simulink model "CSF_Model"  (R2022a)
settings: Solver=ode4  StartTime=0.0  StopTime=10000  FixedStep=0.01  MaxStep=0.1  MinStep=0.01  RelTol=1e-3  AbsTol=1e-6
undefined symbols (not defined in the file): b_EA, E_A0, E_C, E_IEG, E_SAS, E_V, E_VEN, f_ECS, f_SPI, k_m, P_ECS0, P_OLS, P_SLS, P_SPI0, P_SSS, pi_C0, pi_ECS0, Q_CSF, R_A0, R_AG, R_BBB, R_C0, R_CMC, R_CP, R_ECS, R_FM, R_IEGH, R_IEGL, R_PAS, R_PCS, R_PNS, R_SAS, R_SPI, R_V0, R_VEN, R_VEN0, sigbuilder_block, V_A0, V_Afree, V_BT_solid, V_C0, V_Cfree, V_ECS0, V_ICS0, V_PAS0, V_PNS0, V_SAS0, V_SPI0, V_T0, V_V0, V_VEN0, V_VEN_free, V_Vfree
libraries: cstblocks x8, dspstat3 x6, simulink x1
settings Model: SnapshotInterval=1  Creator=Administrator  LastModifiedBy=Administrator

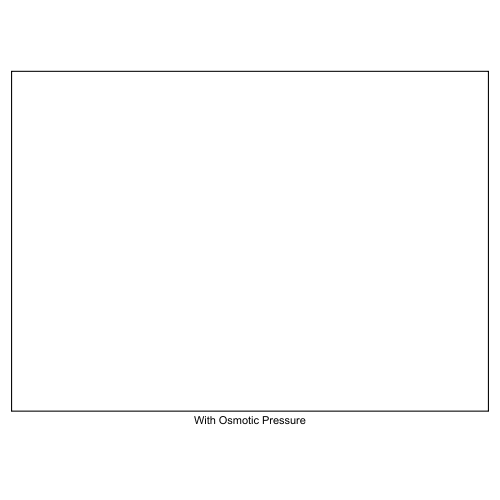
[thumbnail: Simulink's stored preview of the top-level diagram]
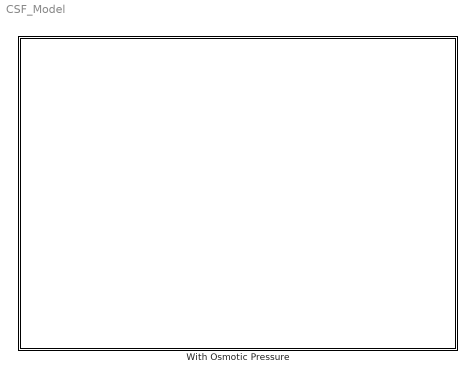
== system CSF_Model ==
  With Osmotic Pressure : Subsystem

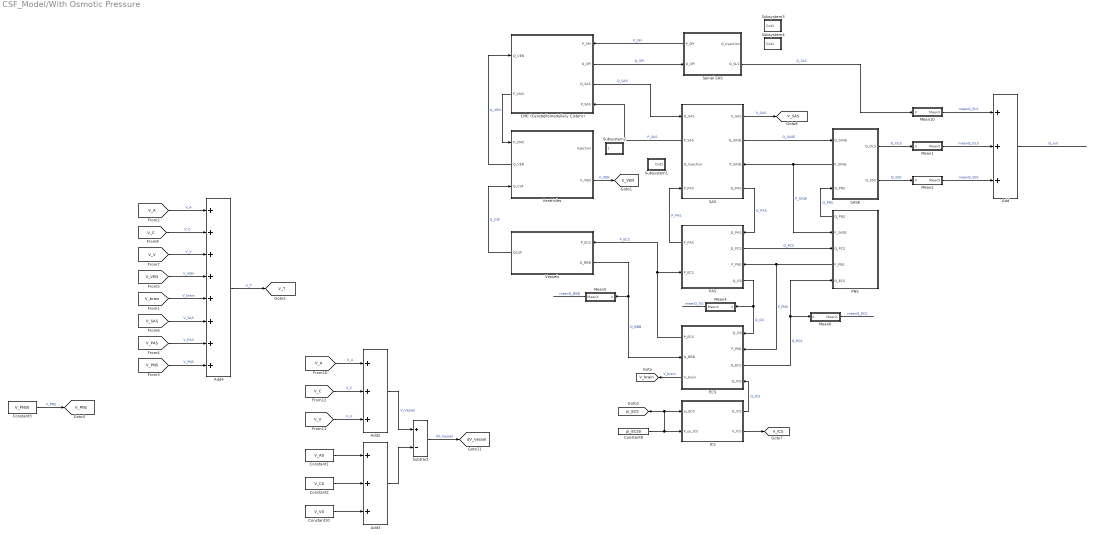
== system CSF_Model/With Osmotic Pressure ==
  Add : Sum  Inputs=+++
  Add2 : Sum  Inputs=+++
  Add3 : Sum  Inputs=+++
  Add4 : Sum  Inputs=++++++++
  CMC (Cerebellomedullary Cistern) : Subsystem
      settings: PortSchema="{\"entries\":[{\"content\":{\"sides\":[{\"content\":{\"connectorIds\":[\"In1\",\"Out3\"]},\"type\":\"ConnectorPlacement.EquallySpacedRectSide\",\"uuid\":\"013a87ed-5019-4cf7-bc7e-b763ecbf40be\"},{\"content\":{\"connectorIds\":[\"In2\",\"Out1\",\"Out2\",\"In3\"],\"side\":\"RIGHT\"},\"type\":\"ConnectorPlacement.EquallySpacedRectSide\",\"uuid\":\"57b2f7c1-58ac-4b82-ab5b-e050e476b33b\"},{\"content\":{\"connectorIds\":[],\"side\":\"TOP\"},\"type\":\"ConnectorPlacement.EquallySpacedRectSide\",\"uuid\":\"da2f9a82-30e0-49d1-9e6c-54ed808c9c6e\"}]},\"type\":\"ConnectorPlacement.EquallySpacedConnector\",\"uuid\":\"bd940c80-8986-43bc-ad7b-1b94db1ac316\"}],\"packageUris\":[\"http://schema.mathworks.com/mf0/Connector/R2020b\"],\"version\":\"1.0\"}"
  Constant1 : Constant  Value=V_A0
  Constant10 : Constant  Value=V_V0
  Constant2 : Constant  Value=V_C0
  Constant3 : Constant  Value=V_PNS0
  Constant8 : Constant  Value=pi_ECS0
  ECS : Subsystem
      settings: PortSchema="{\"entries\":[{\"content\":{\"sides\":[{\"content\":{\"connectorIds\":[\"Out2\",\"In1\",\"Out3\"]},\"type\":\"ConnectorPlacement.EquallySpacedRectSide\",\"uuid\":\"d1e0d4a5-d76a-43bf-98e1-ed8a33587d94\"},{\"content\":{\"connectorIds\":[\"In2\",\"Out1\",\"In3\",\"In4\"],\"side\":\"RIGHT\"},\"type\":\"ConnectorPlacement.EquallySpacedRectSide\",\"uuid\":\"a93046bb-1935-4fcc-a858-465d9e877f86\"},{\"content\":{\"connectorIds\":[],\"side\":\"TOP\"},\"type\":\"ConnectorPlacement.EquallySpacedRectSide\",\"uuid\":\"8ff1877f-8428-43f4-bdc2-a7f63dce98e3\"}]},\"type\":\"ConnectorPlacement.EquallySpacedConnector\",\"uuid\":\"3a5fbfdf-c4c7-43cd-80c3-39c50f2079ec\"}],\"packageUris\":[\"http://schema.mathworks.com/mf0/Connector/R2020b\"],\"version\":\"1.0\"}"
  ICS : Subsystem
  Mean1 : Subsystem
  Mean10 : Subsystem
  Mean2 : Subsystem
  Mean4 : Subsystem
  Mean5 : Subsystem
  Mean6 : Subsystem
  PAS : Subsystem
      settings: PortSchema="{\"entries\":[{\"content\":{\"sides\":[{\"content\":{\"connectorIds\":[\"Out3\",\"In1\"]},\"type\":\"ConnectorPlacement.EquallySpacedRectSide\",\"uuid\":\"c2f26e20-6fa7-4bf6-bac3-e1e4e9c4ec58\"},{\"content\":{\"connectorIds\":[\"In2\",\"Out1\",\"In3\",\"Out2\"],\"side\":\"RIGHT\"},\"type\":\"ConnectorPlacement.EquallySpacedRectSide\",\"uuid\":\"ae54b47a-8b10-42ee-b40e-b80c64c909c9\"},{\"content\":{\"connectorIds\":[],\"side\":\"TOP\"},\"type\":\"ConnectorPlacement.EquallySpacedRectSide\",\"uuid\":\"815b1455-9f59-434d-88b0-8812fa628978\"},{\"content\":{\"connectorIds\":[],\"side\":\"BOTTOM\"},\"type\":\"ConnectorPlacement.EquallySpacedRectSide\",\"uuid\":\"6b900877-34b4-4b91-99fd-dbb8757fe9e6\"}]},\"type\":\"ConnectorPlacement.EquallySpacedConnector\",\"uuid\":\"ecef9f3d-643d-4d92-8968-e42d0387bb2a\"}],\"packageUris\":[\"http://schema.mathworks.com/mf0/Connector/R2020b\"],\"version\":\"1.0\"}"
  PNS : Subsystem
      settings: PortSchema="{\"entries\":[{\"content\":{\"sides\":[{\"content\":{\"connectorIds\":[\"Out1\",\"In1\",\"In2\",\"Out2\",\"In3\"]},\"type\":\"ConnectorPlacement.EquallySpacedRectSide\",\"uuid\":\"5fbe6c9d-3498-4146-9f0b-b77779ec6dad\"},{\"content\":{\"connectorIds\":[],\"side\":\"RIGHT\"},\"type\":\"ConnectorPlacement.EquallySpacedRectSide\",\"uuid\":\"fbf01b15-7a9f-409e-af5d-c73289629c2f\"},{\"content\":{\"connectorIds\":[],\"side\":\"TOP\"},\"type\":\"ConnectorPlacement.EquallySpacedRectSide\",\"uuid\":\"84a27698-b118-4183-ac33-cd71cc4704df\"}]},\"type\":\"ConnectorPlacement.EquallySpacedConnector\",\"uuid\":\"3a25198c-4299-4e36-a61d-eed86b0dea68\"}],\"packageUris\":[\"http://schema.mathworks.com/mf0/Connector/R2020b\"],\"version\":\"1.0\"}"
  SAS : Subsystem
      settings: PortSchema="{\"entries\":[{\"content\":{\"sides\":[{\"content\":{\"connectorIds\":[\"In1\",\"Out4\",\"In2\",\"In3\"]},\"type\":\"ConnectorPlacement.EquallySpacedRectSide\",\"uuid\":\"ca5be0dd-e4d9-4d74-8ff5-165f520bee20\"},{\"content\":{\"connectorIds\":[\"Out1\",\"Out2\",\"In4\",\"Out3\"],\"side\":\"RIGHT\"},\"type\":\"ConnectorPlacement.EquallySpacedRectSide\",\"uuid\":\"d1bc81c7-8cba-48bb-8bc1-5472ec1443ad\"},{\"content\":{\"connectorIds\":[],\"side\":\"TOP\"},\"type\":\"ConnectorPlacement.EquallySpacedRectSide\",\"uuid\":\"685eba57-22e9-4397-b0db-5008f2d3101d\"}]},\"type\":\"ConnectorPlacement.EquallySpacedConnector\",\"uuid\":\"2486ab90-8cac-42ad-9c36-b2644eb474f8\"}],\"packageUris\":[\"http://schema.mathworks.com/mf0/Connector/R2020b\"],\"version\":\"1.0\"}"
  SASE : Subsystem
      settings: PortSchema="{\"entries\":[{\"content\":{\"sides\":[{\"content\":{\"connectorIds\":[\"In1\",\"Out3\",\"In2\"]},\"type\":\"ConnectorPlacement.EquallySpacedRectSide\",\"uuid\":\"73239018-6b84-4d1b-a39c-7360c9503bc6\"},{\"content\":{\"connectorIds\":[\"Out1\",\"Out2\"],\"side\":\"RIGHT\"},\"type\":\"ConnectorPlacement.EquallySpacedRectSide\",\"uuid\":\"b723cfc7-fedc-421a-9fba-aa0734355de6\"},{\"content\":{\"connectorIds\":[],\"side\":\"TOP\"},\"type\":\"ConnectorPlacement.EquallySpacedRectSide\",\"uuid\":\"de4b320f-3afa-4cf6-aa90-abae206980c0\"}]},\"type\":\"ConnectorPlacement.EquallySpacedConnector\",\"uuid\":\"1ba6b848-2c16-4613-b6b1-fdcb918bcf69\"}],\"packageUris\":[\"http://schema.mathworks.com/mf0/Connector/R2020b\"],\"version\":\"1.0\"}"
  Spinal SAS : Subsystem
      settings: PortSchema="{\"entries\":[{\"content\":{\"sides\":[{\"content\":{\"connectorIds\":[\"Out2\",\"In1\"]},\"type\":\"ConnectorPlacement.EquallySpacedRectSide\",\"uuid\":\"013a87ed-5019-4cf7-bc7e-b763ecbf40be\"},{\"content\":{\"connectorIds\":[\"In2\",\"Out1\"],\"side\":\"RIGHT\"},\"type\":\"ConnectorPlacement.EquallySpacedRectSide\",\"uuid\":\"57b2f7c1-58ac-4b82-ab5b-e050e476b33b\"},{\"content\":{\"connectorIds\":[],\"side\":\"TOP\"},\"type\":\"ConnectorPlacement.EquallySpacedRectSide\",\"uuid\":\"da2f9a82-30e0-49d1-9e6c-54ed808c9c6e\"}]},\"type\":\"ConnectorPlacement.EquallySpacedConnector\",\"uuid\":\"bd940c80-8986-43bc-ad7b-1b94db1ac316\"}],\"packageUris\":[\"http://schema.mathworks.com/mf0/Connector/R2020b\"],\"version\":\"1.0\"}"
  Subsystem1 : Subsystem
  Subsystem2 : Subsystem
  Subsystem3 : Subsystem
  Subsystem4 : Subsystem
  Subtract : Sum  Inputs=+-
  Ventricles : Subsystem
      settings: PortSchema="{\"entries\":[{\"content\":{\"sides\":[{\"content\":{\"connectorIds\":[\"In1\",\"Out2\",\"In2\"]},\"type\":\"ConnectorPlacement.EquallySpacedRectSide\",\"uuid\":\"013a87ed-5019-4cf7-bc7e-b763ecbf40be\"},{\"content\":{\"connectorIds\":[\"In3\",\"Out1\"],\"side\":\"RIGHT\"},\"type\":\"ConnectorPlacement.EquallySpacedRectSide\",\"uuid\":\"57b2f7c1-58ac-4b82-ab5b-e050e476b33b\"},{\"content\":{\"connectorIds\":[],\"side\":\"TOP\"},\"type\":\"ConnectorPlacement.EquallySpacedRectSide\",\"uuid\":\"da2f9a82-30e0-49d1-9e6c-54ed808c9c6e\"}]},\"type\":\"ConnectorPlacement.EquallySpacedConnector\",\"uuid\":\"bd940c80-8986-43bc-ad7b-1b94db1ac316\"}],\"packageUris\":[\"http://schema.mathworks.com/mf0/Connector/R2020b\"],\"version\":\"1.0\"}"
  Vessels : Subsystem
      settings: PortSchema="{\"entries\":[{\"content\":{\"sides\":[{\"content\":{\"connectorIds\":[\"Out2\"]},\"type\":\"ConnectorPlacement.EquallySpacedRectSide\",\"uuid\":\"02216f8d-b656-405c-ace7-fa57996d1b51\"},{\"content\":{\"connectorIds\":[\"In1\",\"Out1\"],\"side\":\"RIGHT\"},\"type\":\"ConnectorPlacement.EquallySpacedRectSide\",\"uuid\":\"1efca463-a03b-437d-a556-a9f9cadbd1b9\"},{\"content\":{\"connectorIds\":[],\"side\":\"TOP\"},\"type\":\"ConnectorPlacement.EquallySpacedRectSide\",\"uuid\":\"405cde4e-e8e7-4444-912c-c8c68c2302e6\"}]},\"type\":\"ConnectorPlacement.EquallySpacedConnector\",\"uuid\":\"ec00ee8b-baba-493b-8b97-ad2027431ac2\"}],\"packageUris\":[\"http://schema.mathworks.com/mf0/Connector/R2020b\"],\"version\":\"1.0\"}"
  tag scope: V_ICS=global, V_PNS=global, V_SAS=global, V_T=global, V_VEN=global, V_brain=global, dV_Vessel=global, pi_ECS=global
  wires:
  SAS/1(V_SAS) -> [V_SAS]  "V_SAS"
  Mean1/1(MeanX) -> Add/2  "meanQ_OLS"
  ECS/2(V_brain) -> [V_brain]  "V_brain"
  ICS/1(Q_ICS) -> ECS/2(Q_ICS)  "Q_ICS"
  ICS/2(V_ICS) -> [V_ICS]
  SASE/2(Q_SSS) -> Mean2/1(X)  "Q_SSS"
  Mean2/1(MeanX) -> Add/3  "meanQ_SSS"
  ECS/3(P_ECS) -> PAS/1(P_ECS), Vessels/1(P_ECS)  "P_ECS"
  ECS/1(Q_ECS) -> Mean6/1(X), PNS/3(Q_ECS)  "Q_ECS"
  SASE/1(Q_OLS) -> Mean1/1(X)  "Q_OLS"
  PAS/3(P_PAS) -> SAS/3(P_PAS)  "P_PAS"
  PNS/1(Q_PNS) -> SASE/2(Q_PNS)  "Q_PNS"
  PAS/2(Q_GS) -> Mean4/1(X), ECS/4(Q_GS)  "Q_GS"
  PNS/2(P_PNS) -> ECS/3(P_PNS), PAS/3(P_PNS)  "P_PNS"
  PAS/1(Q_PCS) -> PNS/2(Q_PCS)  "Q_PCS"
  Ventricles/1(V_VEN) -> [V_VEN]  "V_VEN"
  SASE/3(P_SASE) -> PNS/1(P_SASE), SAS/4(P_SASE)  "P_SASE"
  Add/1 -> ?  "Q_out"
  Mean6/1(MeanX) -> ?  "meanQ_ECS"
  Constant8/1 -> [pi_ECS], ICS/1(pi_ECS), ICS/2(P_os_ICS)
  Vessels/1(Q_BBB) -> ECS/1(Q_BBB), Mean5/1(X)  "Q_BBB"
  Vessels/2(QCSF) -> Ventricles/2(Q_CSF)  "Q_CSF"
  Spinal SAS/1(Q_SLS) -> Mean10/1(X)  "Q_SLS"
  Mean10/1(MeanX) -> Add/1  "meanQ_SLS"
  SAS/4(P_SAS) -> CMC (Cerebellomedullary Cistern)/3(P_SAS)  "P_SAS"
  CMC (Cerebellomedullary Cistern)/2(Q_SAS) -> SAS/1(Q_SAS)  "Q_SAS"
  Add4/1 -> [V_T]  "V_T"
  [V_C] -> Add4/2  "V_C"
  [V_SAS] -> Add4/6  "V_SAS"
  [V_VEN] -> Add4/4  "V_VEN"
  [V_V] -> Add4/3  "V_V"
  [V_PNS] -> Add4/8  "V_PNS"
  [V_A] -> Add4/1  "V_A"
  [V_brain] -> Add4/5  "V_brain"
  [V_PAS] -> Add4/7  "V_PAS"
  Mean4/1(MeanX) -> ?  "meanQ_GS"
  SAS/3(Q_PAS) -> PAS/2(Q_PAS)  "Q_PAS"
  SAS/2(Q_SASE) -> SASE/1(Q_SASE)  "Q_SASE"
  Mean5/1(MeanX) -> ?  "meanQ_BBB"
  Constant3/1 -> [V_PNS]  "V_PNS"
  Spinal SAS/2(P_SPI) -> CMC (Cerebellomedullary Cistern)/2(P_SPI)  "P_SPI"
  CMC (Cerebellomedullary Cistern)/1(Q_SPI) -> Spinal SAS/1(Q_SPI)  "Q_SPI"
  [V_C] -> Add2/2  "V_C"
  [V_V] -> Add2/3  "V_V"
  [V_A] -> Add2/1  "V_A"
  Constant1/1 -> Add3/1
  Constant2/1 -> Add3/2
  Constant10/1 -> Add3/3
  Subtract/1 -> [dV_Vessel]  "dV_Vessel"
  Add2/1 -> Subtract/1  "V_Vessel"
  Add3/1 -> Subtract/2
  Ventricles/2(Q_VEN) -> CMC (Cerebellomedullary Cistern)/1(Q_VEN)  "Q_VEN"
  CMC (Cerebellomedullary Cistern)/3(P_CMC) -> Ventricles/1(P_CMC)

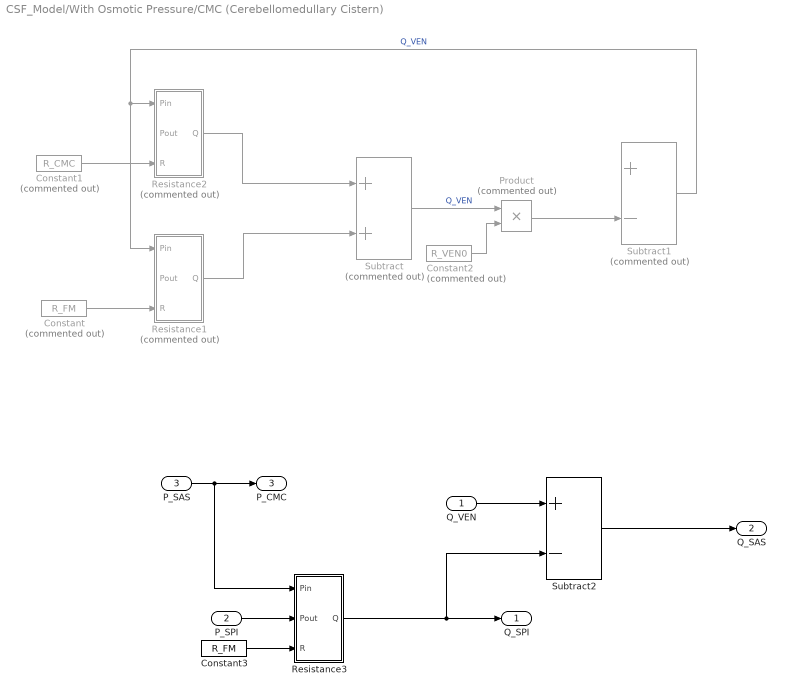
== system CSF_Model/With Osmotic Pressure/CMC (Cerebellomedullary Cistern) ==
  Q_VEN : Inport
  P_SPI : Inport  Port=2
  P_SAS : Inport  Port=3
  Constant : Constant  Commented=on  Value=R_FM
  Constant1 : Constant  Commented=on  Value=R_CMC
  Constant2 : Constant  Commented=on  Value=R_VEN0
  Constant3 : Constant  Value=R_FM
  Product : Product  Commented=on
  Resistance1 : Subsystem  Commented=on
  Resistance2 : Subsystem  Commented=on
  Resistance3 : Subsystem
  Subtract : Sum  Commented=on
  Subtract1 : Sum  Commented=on  Inputs=+-
  Subtract2 : Sum  Inputs=+-
  Q_SPI : Outport
  Q_SAS : Outport  Port=2
  P_CMC : Outport  Port=3
  wires:
  Constant/1 -> Resistance1/3(R)
  Resistance1/1(Q) -> Subtract/2
  Constant1/1 -> Resistance2/3(R)
  Resistance2/1(Q) -> Subtract/1
  Subtract/1 -> Product/1  "Q_VEN"
  Constant2/1 -> Product/2
  Product/1 -> Subtract1/2
  Subtract1/1 -> Resistance1/1(Pin), Resistance2/1(Pin)  "Q_VEN"
  P_SAS/1 -> Resistance3/1(Pin), P_CMC/1
  P_SPI/1 -> Resistance3/2(Pout)
  Constant3/1 -> Resistance3/3(R)
  Resistance3/1(Q) -> Subtract2/2, Q_SPI/1
  Q_VEN/1 -> Subtract2/1
  Subtract2/1 -> Q_SAS/1

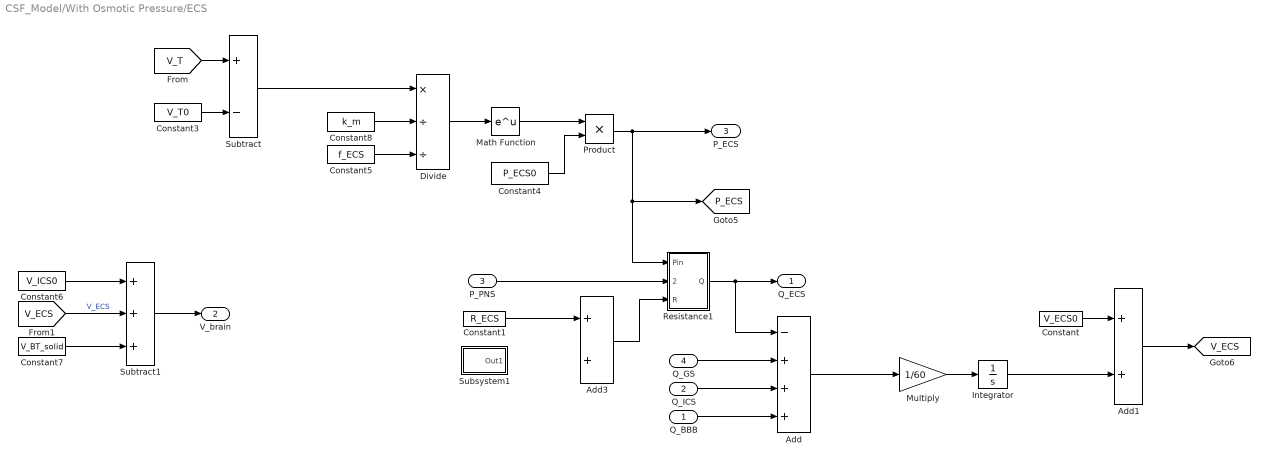
== system CSF_Model/With Osmotic Pressure/ECS ==
  Q_BBB : Inport
  Q_ICS : Inport  Port=2
  P_PNS : Inport  Port=3
  Q_GS : Inport  Port=4
  Add : Sum  Inputs=-+++
  Add1 : Sum
  Add3 : Sum
  Constant : Constant  Value=V_ECS0
  Constant1 : Constant  Value=R_ECS
  Constant3 : Constant  Value=V_T0
  Constant4 : Constant  Value=P_ECS0
  Constant5 : Constant  Value=f_ECS
  Constant6 : Constant  Value=V_ICS0
  Constant7 : Constant  Value=V_BT_solid
  Constant8 : Constant  Value=k_m
  Divide : Product  Inputs=*//
  Integrator : Integrator
  Math Function : Math
  Multiply : Gain  Gain=1/60
  Product : Product
  Resistance1 : Subsystem
  Subsystem1 : Subsystem
  Subtract : Sum  Inputs=+-
  Subtract1 : Sum  Inputs=+++
  Q_ECS : Outport
  V_brain : Outport  Port=2
  P_ECS : Outport  Port=3
  tag scope: P_ECS=global, V_ECS=global
  wires:
  Add3/1 -> Resistance1/3(R)
  Resistance1/1(Q) -> Add/1, Q_ECS/1
  Constant1/1 -> Add3/1
  P_PNS/1 -> Resistance1/2(Pout)
  Add1/1 -> [V_ECS]
  Add/1 -> Multiply/1
  Q_ICS/1 -> Add/3
  Q_GS/1 -> Add/2
  Product/1 -> Resistance1/1(Pin), [P_ECS], P_ECS/1
  Q_BBB/1 -> Add/4
  Multiply/1 -> Integrator/1
  Constant5/1 -> Divide/3
  Constant8/1 -> Divide/2
  Math Function/1 -> Product/1
  Divide/1 -> Math Function/1
  Constant4/1 -> Product/2
  Integrator/1 -> Add1/2
  Constant/1 -> Add1/1
  [V_T] -> Subtract/1
  Constant3/1 -> Subtract/2
  Constant6/1 -> Subtract1/1
  [V_ECS] -> Subtract1/2  "V_ECS"
  Subtract1/1 -> V_brain/1
  Constant7/1 -> Subtract1/3
  Subtract/1 -> Divide/1

== system CSF_Model/With Osmotic Pressure/ICS ==
  pi_ECS : Inport
  P_os_ICS : Inport  Port=2
  Add : Sum
  Constant2 : Constant  Value=V_ICS0
  Constant3 : Constant
  Integrator : Integrator
  Multiply : Gain  Gain=-1
  Multiply1 : Gain  Gain=-1
  Multiply2 : Gain  Gain=-1
  Resistance1 : Subsystem
  Q_ICS : Outport
  V_ICS : Outport  Port=2
  wires:
  Add/1 -> V_ICS/1
  Constant2/1 -> Add/2
  Integrator/1 -> Add/1
  Multiply/1 -> Integrator/1
  Resistance1/1(Q) -> Q_ICS/1, Multiply/1
  pi_ECS/1 -> Multiply1/1
  P_os_ICS/1 -> Multiply2/1
  Multiply1/1 -> Resistance1/1(Pin)
  Multiply2/1 -> Resistance1/2(Pout)
  Constant3/1 -> Resistance1/3(R)

== system CSF_Model/With Osmotic Pressure/Mean1 ==
  X : Inport
  Constant : Constant  Value=0.1
  Moving Average : dspstat3/Moving Average  Method=Sliding window  ForgettingFactorPort=off  SpecifyWindowLength=on  WindowLength=1  ForgettingFactor=0.9  SimulateUsing=Code generation
  Product : Product
  Step : Step  Time=10  SampleTime=0
  Varying Lowpass Filter : cstblocks/Linear Parameter Varying/Varying Lowpass Filter  N=1
  MeanX : Outport
  wires:
  Constant/1 -> Varying Lowpass Filter/2
  X/1 -> Product/2
  Moving Average/1 -> Varying Lowpass Filter/1
  Product/1 -> Moving Average/1
  Step/1 -> Product/1
  Varying Lowpass Filter/1 -> MeanX/1

== system CSF_Model/With Osmotic Pressure/Mean10 ==
  X : Inport
  Constant : Constant  Value=0.1
  Moving Average : dspstat3/Moving Average  Method=Sliding window  ForgettingFactorPort=off  SpecifyWindowLength=on  WindowLength=1  ForgettingFactor=0.9  SimulateUsing=Code generation
  Product : Product
  Step : Step  Time=10  SampleTime=0
  Varying Lowpass Filter : cstblocks/Linear Parameter Varying/Varying Lowpass Filter  N=1
  MeanX : Outport
  wires:
  Constant/1 -> Varying Lowpass Filter/2
  X/1 -> Product/2
  Moving Average/1 -> Varying Lowpass Filter/1
  Product/1 -> Moving Average/1
  Step/1 -> Product/1
  Varying Lowpass Filter/1 -> MeanX/1

== system CSF_Model/With Osmotic Pressure/Mean2 ==
  X : Inport
  Constant : Constant  Value=0.1
  Moving Average : dspstat3/Moving Average  Method=Sliding window  ForgettingFactorPort=off  SpecifyWindowLength=on  WindowLength=1  ForgettingFactor=0.9  SimulateUsing=Code generation
  Product : Product
  Step : Step  Time=10  SampleTime=0
  Varying Lowpass Filter : cstblocks/Linear Parameter Varying/Varying Lowpass Filter  N=1
  MeanX : Outport
  wires:
  Constant/1 -> Varying Lowpass Filter/2
  X/1 -> Product/2
  Moving Average/1 -> Varying Lowpass Filter/1
  Product/1 -> Moving Average/1
  Step/1 -> Product/1
  Varying Lowpass Filter/1 -> MeanX/1

== system CSF_Model/With Osmotic Pressure/Mean4 ==
  X : Inport
  Constant : Constant  Value=0.1
  Constant1 : Constant  Value=0.1
  Moving Average1 : dspstat3/Moving Average  Method=Sliding window  ForgettingFactorPort=off  SpecifyWindowLength=on  WindowLength=1  ForgettingFactor=0.9  SimulateUsing=Code generation
  Product : Product
  Step : Step  Time=10  SampleTime=0
  Varying Lowpass Filter : cstblocks/Linear Parameter Varying/Varying Lowpass Filter  N=1
  Varying Lowpass Filter1 : cstblocks/Linear Parameter Varying/Varying Lowpass Filter  N=1
  MeanX : Outport
  wires:
  Constant/1 -> Varying Lowpass Filter/2
  X/1 -> Product/2
  Product/1 -> Moving Average1/1
  Step/1 -> Product/1
  Varying Lowpass Filter/1 -> Varying Lowpass Filter1/1
  Moving Average1/1 -> Varying Lowpass Filter/1
  Constant1/1 -> Varying Lowpass Filter1/2
  Varying Lowpass Filter1/1 -> MeanX/1

== system CSF_Model/With Osmotic Pressure/Mean5 ==
  X : Inport
  Constant : Constant  Value=0.1
  Moving Average : dspstat3/Moving Average  Method=Sliding window  ForgettingFactorPort=off  SpecifyWindowLength=on  WindowLength=1  ForgettingFactor=0.9  SimulateUsing=Code generation
  Product : Product
  Step : Step  Time=10  SampleTime=0
  Varying Lowpass Filter : cstblocks/Linear Parameter Varying/Varying Lowpass Filter  N=1
  MeanX : Outport
  wires:
  Constant/1 -> Varying Lowpass Filter/2
  X/1 -> Product/2
  Moving Average/1 -> Varying Lowpass Filter/1
  Product/1 -> Moving Average/1
  Step/1 -> Product/1
  Varying Lowpass Filter/1 -> MeanX/1

== system CSF_Model/With Osmotic Pressure/Mean6 ==
  X : Inport
  Constant : Constant  Value=0.1
  Moving Average : dspstat3/Moving Average  Method=Sliding window  ForgettingFactorPort=off  SpecifyWindowLength=on  WindowLength=1  ForgettingFactor=0.9  SimulateUsing=Code generation
  Product : Product
  Step : Step  Time=10  SampleTime=0
  Varying Lowpass Filter : cstblocks/Linear Parameter Varying/Varying Lowpass Filter  N=1
  MeanX : Outport
  wires:
  Constant/1 -> Varying Lowpass Filter/2
  X/1 -> Product/2
  Moving Average/1 -> Varying Lowpass Filter/1
  Product/1 -> Moving Average/1
  Step/1 -> Product/1
  Varying Lowpass Filter/1 -> MeanX/1

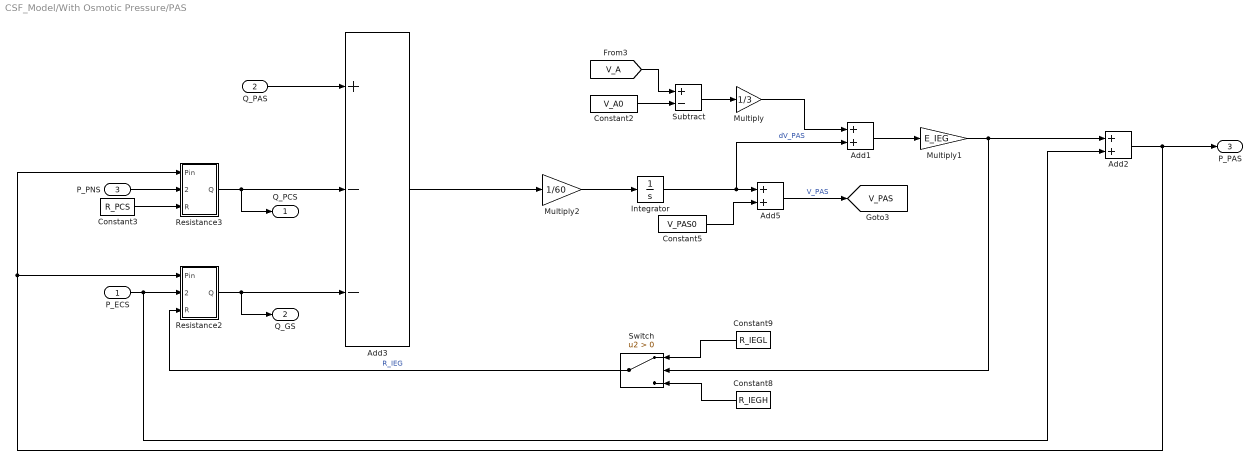
== system CSF_Model/With Osmotic Pressure/PAS ==
  P_ECS : Inport
  Q_PAS : Inport  Port=2
  P_PNS : Inport  Port=3
  Add1 : Sum
  Add2 : Sum
  Add3 : Sum  Inputs=+--
  Add5 : Sum
  Constant2 : Constant  Value=V_A0
  Constant3 : Constant  Value=R_PCS
  Constant5 : Constant  Value=V_PAS0
  Constant8 : Constant  Value=R_IEGH
  Constant9 : Constant  Value=R_IEGL
  Integrator : Integrator
  Multiply : Gain  Gain=1/3
  Multiply1 : Gain  Gain=E_IEG
  Multiply2 : Gain  Gain=1/60
  Resistance2 : Subsystem
  Resistance3 : Subsystem
  Subtract : Sum  Inputs=+-
  Switch : Switch  Criteria=u2 > Threshold  SaturateOnIntegerOverflow=off  InputSameDT=off
  Q_PCS : Outport
  Q_GS : Outport  Port=2
  P_PAS : Outport  Port=3
  tag scope: V_PAS=global
  wires:
  Multiply1/1 -> Switch/2, Add2/1
  Constant9/1 -> Switch/1
  Resistance2/1(Q) -> Add3/3, Q_GS/1
  Resistance3/1(Q) -> Q_PCS/1, Add3/2
  Constant3/1 -> Resistance3/3(R)
  Q_PAS/1 -> Add3/1
  Add3/1 -> Multiply2/1
  Integrator/1 -> Add1/2, Add5/1  "dV_PAS"
  Constant5/1 -> Add5/2
  Add1/1 -> Multiply1/1
  Add2/1 -> P_PAS/1, Resistance3/1(Pin), Resistance2/1(Pin)
  [V_A] -> Subtract/1
  P_PNS/1 -> Resistance3/2(Pout)
  Add5/1 -> [V_PAS]  "V_PAS"
  Subtract/1 -> Multiply/1
  Constant2/1 -> Subtract/2
  P_ECS/1 -> Add2/2, Resistance2/2(Pout)
  Constant8/1 -> Switch/3
  Multiply2/1 -> Integrator/1
  Multiply/1 -> Add1/1
  Switch/1 -> Resistance2/3(R)  "R_IEG"

== system CSF_Model/With Osmotic Pressure/PNS ==
  P_SASE : Inport
  Q_PCS : Inport  Port=2
  Q_ECS : Inport  Port=3
  Add : Sum
  Add1 : Sum
  Constant : Constant  Value=R_PNS
  Product : Product
  Q_PNS : Outport
  P_PNS : Outport  Port=2
  tag scope: P_PNS=global
  wires:
  Q_PCS/1 -> Add/1
  Product/1 -> Add1/2
  Add1/1 -> [P_PNS], P_PNS/1  "P_PNS"
  Constant/1 -> Product/1
  P_SASE/1 -> Add1/1
  Add/1 -> Product/2, Q_PNS/1  "Q_PCS"
  Q_ECS/1 -> Add/2

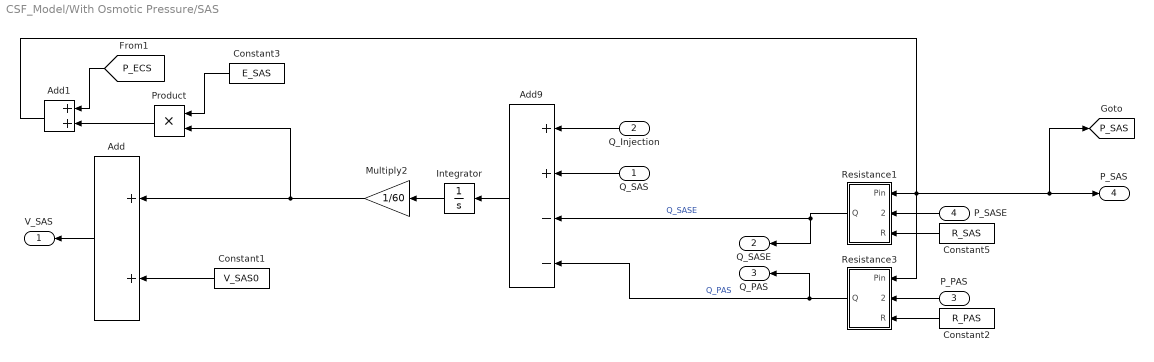
== system CSF_Model/With Osmotic Pressure/SAS ==
  Q_SAS : Inport
  Q_Injection : Inport  Port=2
  P_PAS : Inport  Port=3
  P_SASE : Inport  Port=4
  Add : Sum
  Add1 : Sum
  Add9 : Sum  Inputs=++--
  Constant1 : Constant  Value=V_SAS0
  Constant2 : Constant  Value=R_PAS
  Constant3 : Constant  Value=E_SAS
  Constant5 : Constant  Value=R_SAS
  Integrator : Integrator
  Multiply2 : Gain  Gain=1/60
  Product : Product
  Resistance1 : Subsystem
  Resistance3 : Subsystem
  V_SAS : Outport
  Q_SASE : Outport  Port=2
  Q_PAS : Outport  Port=3
  P_SAS : Outport  Port=4
  tag scope: P_SAS=global
  wires:
  Resistance3/1(Q) -> Add9/4, Q_PAS/1  "Q_PAS"
  Resistance1/1(Q) -> Add9/3, Q_SASE/1  "Q_SASE"
  Q_Injection/1 -> Add9/1
  Q_SAS/1 -> Add9/2
  Constant2/1 -> Resistance3/3(R)
  P_PAS/1 -> Resistance3/2(Pout)
  P_SASE/1 -> Resistance1/2(Pout)
  Constant5/1 -> Resistance1/3(R)
  Add9/1 -> Integrator/1
  Integrator/1 -> Multiply2/1
  Constant1/1 -> Add/2
  Add/1 -> V_SAS/1
  Constant3/1 -> Product/1
  Product/1 -> Add1/2
  [P_ECS] -> Add1/1
  Add1/1 -> Resistance3/1(Pin), [P_SAS], P_SAS/1, Resistance1/1(Pin)
  Multiply2/1 -> Product/2, Add/1

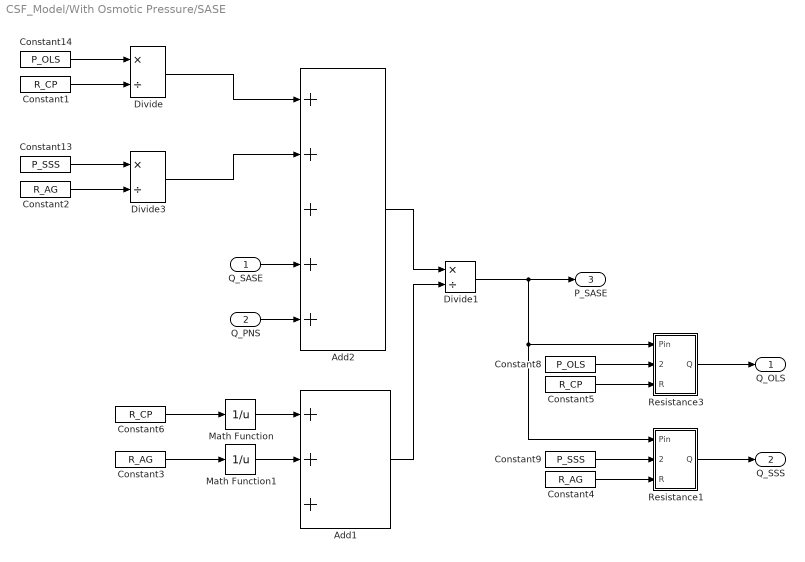
== system CSF_Model/With Osmotic Pressure/SASE ==
  Q_SASE : Inport
  Q_PNS : Inport  Port=2
  Add1 : Sum  Inputs=+++
  Add2 : Sum  Inputs=+++++
  Constant1 : Constant  Value=R_CP
  Constant13 : Constant  Value=P_SSS
  Constant14 : Constant  Value=P_OLS
  Constant2 : Constant  Value=R_AG
  Constant3 : Constant  Value=R_AG
  Constant4 : Constant  Value=R_AG
  Constant5 : Constant  Value=R_CP
  Constant6 : Constant  Value=R_CP
  Constant8 : Constant  Value=P_OLS
  Constant9 : Constant  Value=P_SSS
  Divide : Product  Inputs=*/
  Divide1 : Product  Inputs=*/
  Divide3 : Product  Inputs=*/
  Math Function : Math  Operator=reciprocal
  Math Function1 : Math  Operator=reciprocal
  Resistance1 : Subsystem
  Resistance3 : Subsystem
  Q_OLS : Outport
  Q_SSS : Outport  Port=2
  P_SASE : Outport  Port=3
  wires:
  Constant14/1 -> Divide/1
  Constant1/1 -> Divide/2
  Constant13/1 -> Divide3/1
  Constant2/1 -> Divide3/2
  Divide/1 -> Add2/1
  Divide3/1 -> Add2/2
  Q_SASE/1 -> Add2/4
  Q_PNS/1 -> Add2/5
  Add2/1 -> Divide1/1
  Constant6/1 -> Math Function/1
  Constant3/1 -> Math Function1/1
  Math Function/1 -> Add1/1
  Math Function1/1 -> Add1/2
  Add1/1 -> Divide1/2
  Divide1/1 -> Resistance1/1(Pin), Resistance3/1(Pin), P_SASE/1
  Resistance3/1(Q) -> Q_OLS/1
  Constant5/1 -> Resistance3/3(R)
  Constant8/1 -> Resistance3/2(Pout)
  Resistance1/1(Q) -> Q_SSS/1
  Constant9/1 -> Resistance1/2(Pout)
  Constant4/1 -> Resistance1/3(R)

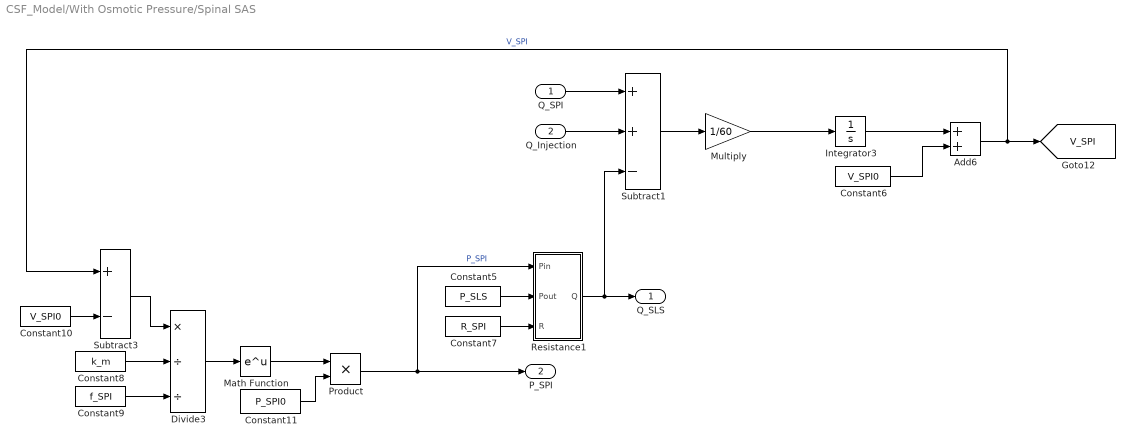
== system CSF_Model/With Osmotic Pressure/Spinal SAS ==
  Q_SPI : Inport
  Q_Injection : Inport  Port=2
  Add6 : Sum
  Constant10 : Constant  Value=V_SPI0
  Constant11 : Constant  Value=P_SPI0
  Constant5 : Constant  Value=P_SLS
  Constant6 : Constant  Value=V_SPI0
  Constant7 : Constant  Value=R_SPI
  Constant8 : Constant  Value=k_m
  Constant9 : Constant  Value=f_SPI
  Divide3 : Product  Inputs=*//
  Integrator3 : Integrator
  Math Function : Math
  Multiply : Gain  Gain=1/60
  Product : Product
  Resistance1 : Subsystem
  Subtract1 : Sum  Inputs=++-
  Subtract3 : Sum  Inputs=+-
  Q_SLS : Outport
  P_SPI : Outport  Port=2
  tag scope: V_SPI=global
  wires:
  Constant6/1 -> Add6/2
  Add6/1 -> [V_SPI], Subtract3/1  "V_SPI"
  Product/1 -> P_SPI/1, Resistance1/1(Pin)  "P_SPI"
  Q_Injection/1 -> Subtract1/2
  Q_SPI/1 -> Subtract1/1
  Constant5/1 -> Resistance1/2(Pout)
  Constant7/1 -> Resistance1/3(R)
  Resistance1/1(Q) -> Q_SLS/1, Subtract1/3
  Subtract1/1 -> Multiply/1
  Integrator3/1 -> Add6/1
  Multiply/1 -> Integrator3/1
  Divide3/1 -> Math Function/1
  Constant8/1 -> Divide3/2
  Subtract3/1 -> Divide3/1
  Constant9/1 -> Divide3/3
  Constant11/1 -> Product/2
  Math Function/1 -> Product/1
  Constant10/1 -> Subtract3/2

== system CSF_Model/With Osmotic Pressure/Subsystem1 ==
  Signal Builder : Subsystem  Tag=STV Subsys  LoadFcn=sigbuilder_block('load');  StartFcn=sigbuilder_block('start');  StopFcn=sigbuilder_block('stop');  ClipboardFcn=sigbuilder_block('clipboard');  mask(Sigbuilder block){tuvar=[0:10]}
      mask help: Simulink:masks:SigbuilderBlock_MD
      mask init:
      | if ~strcmp(get_param(bdroot(gcbh),'SimulationStatus'),'stopped') tuvar = sigbuilder_block('maskInit'); end
      settings: CopyFcn=sigbuilder_block('copy');  DeleteFcn=sigbuilder_block('delete');  ModelCloseFcn=sigbuilder_block('modelClose');  PreSaveFcn=sigbuilder_block('preSave');  PauseFcn=sigbuilder_block('pause');  ContinueFcn=sigbuilder_block('continue');  NameChangeFcn=sigbuilder_block('namechange');  OpenFcn=sigbuilder_block('open',[324.75 228 550.5 399.75 ]);  CloseFcn=sigbuilder_block('close');
      mask Display: plot(0, 0, 100, 100,[2, 2, 32, 32, 2], [68, 8, 8, 68, 68],[32, 2], [38, 38], [32, 19, 2],[53, 60, 44], [32, 17, 17, 2],[16, 16, 31, 31]);txt = getActiveGroup(gcbh);text(2, 100, txt,'verticalAlignment', 'top');
  Out1 : Outport
  wires:
  Signal Builder/1(Signal 1) -> Out1/1

== system CSF_Model/With Osmotic Pressure/Subsystem2 ==
  Signal Builder : Subsystem  Tag=STV Subsys  LoadFcn=sigbuilder_block('load');  StartFcn=sigbuilder_block('start');  StopFcn=sigbuilder_block('stop');  ClipboardFcn=sigbuilder_block('clipboard');  mask(Sigbuilder block){tuvar=[0:10]}
      mask help: Simulink:masks:SigbuilderBlock_MD
      mask init:
      | if ~strcmp(get_param(bdroot(gcbh),'SimulationStatus'),'stopped') tuvar = sigbuilder_block('maskInit'); end
      settings: CopyFcn=sigbuilder_block('copy');  DeleteFcn=sigbuilder_block('delete');  ModelCloseFcn=sigbuilder_block('modelClose');  PreSaveFcn=sigbuilder_block('preSave');  PauseFcn=sigbuilder_block('pause');  ContinueFcn=sigbuilder_block('continue');  NameChangeFcn=sigbuilder_block('namechange');  OpenFcn=sigbuilder_block('open',[324.75 228 550.5 399.75 ]);  CloseFcn=sigbuilder_block('close');
      mask Display: plot(0, 0, 100, 100,[2, 2, 32, 32, 2], [68, 8, 8, 68, 68],[32, 2], [38, 38], [32, 19, 2],[53, 60, 44], [32, 17, 17, 2],[16, 16, 31, 31]);txt = getActiveGroup(gcbh);text(2, 100, txt,'verticalAlignment', 'top');
  Injection : Outport
  wires:
  Signal Builder/1(Signal 1) -> Injection/1

== system CSF_Model/With Osmotic Pressure/Subsystem3 ==
  Signal Builder : Subsystem  Tag=STV Subsys  LoadFcn=sigbuilder_block('load');  StartFcn=sigbuilder_block('start');  StopFcn=sigbuilder_block('stop');  ClipboardFcn=sigbuilder_block('clipboard');  mask(Sigbuilder block){tuvar=[0:10]}
      mask help: Simulink:masks:SigbuilderBlock_MD
      mask init:
      | if ~strcmp(get_param(bdroot(gcbh),'SimulationStatus'),'stopped') tuvar = sigbuilder_block('maskInit'); end
      settings: CopyFcn=sigbuilder_block('copy');  DeleteFcn=sigbuilder_block('delete');  ModelCloseFcn=sigbuilder_block('modelClose');  PreSaveFcn=sigbuilder_block('preSave');  PauseFcn=sigbuilder_block('pause');  ContinueFcn=sigbuilder_block('continue');  NameChangeFcn=sigbuilder_block('namechange');  OpenFcn=sigbuilder_block('open',[324.75 228 550.5 399.75 ]);  CloseFcn=sigbuilder_block('close');
      mask Display: plot(0, 0, 100, 100,[2, 2, 32, 32, 2], [68, 8, 8, 68, 68],[32, 2], [38, 38], [32, 19, 2],[53, 60, 44], [32, 17, 17, 2],[16, 16, 31, 31]);txt = getActiveGroup(gcbh);text(2, 100, txt,'verticalAlignment', 'top');
  Out1 : Outport
  wires:
  Signal Builder/1(Signal 1) -> Out1/1

== system CSF_Model/With Osmotic Pressure/Subsystem4 ==
  Signal Builder : Subsystem  Tag=STV Subsys  LoadFcn=sigbuilder_block('load');  StartFcn=sigbuilder_block('start');  StopFcn=sigbuilder_block('stop');  ClipboardFcn=sigbuilder_block('clipboard');  mask(Sigbuilder block){tuvar=[0:10]}
      mask help: Simulink:masks:SigbuilderBlock_MD
      mask init:
      | if ~strcmp(get_param(bdroot(gcbh),'SimulationStatus'),'stopped') tuvar = sigbuilder_block('maskInit'); end
      settings: CopyFcn=sigbuilder_block('copy');  DeleteFcn=sigbuilder_block('delete');  ModelCloseFcn=sigbuilder_block('modelClose');  PreSaveFcn=sigbuilder_block('preSave');  PauseFcn=sigbuilder_block('pause');  ContinueFcn=sigbuilder_block('continue');  NameChangeFcn=sigbuilder_block('namechange');  OpenFcn=sigbuilder_block('open',[324.75 228 550.5 399.75 ]);  CloseFcn=sigbuilder_block('close');
      mask Display: plot(0, 0, 100, 100,[2, 2, 32, 32, 2], [68, 8, 8, 68, 68],[32, 2], [38, 38], [32, 19, 2],[53, 60, 44], [32, 17, 17, 2],[16, 16, 31, 31]);txt = getActiveGroup(gcbh);text(2, 100, txt,'verticalAlignment', 'top');
  Out1 : Outport
  wires:
  Signal Builder/1(Signal 1) -> Out1/1

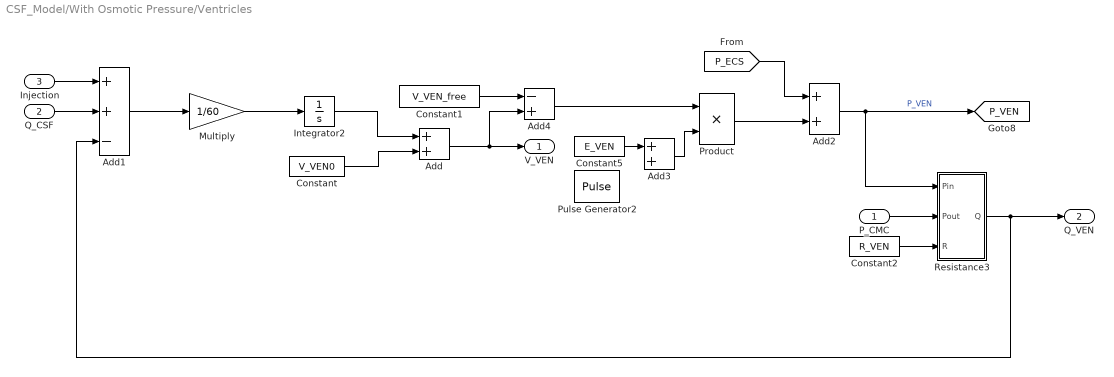
== system CSF_Model/With Osmotic Pressure/Ventricles ==
  P_CMC : Inport
  Q_CSF : Inport  Port=2
  Injection : Inport  Port=3
  Add : Sum
  Add1 : Sum  Inputs=++-
  Add2 : Sum
  Add3 : Sum
  Add4 : Sum  Inputs=-+
  Constant : Constant  Value=V_VEN0
  Constant1 : Constant  Value=V_VEN_free
  Constant2 : Constant  Value=R_VEN
  Constant5 : Constant  Value=E_VEN
  Integrator2 : Integrator
  Multiply : Gain  Gain=1/60
  Product : Product
  Pulse Generator2 : DiscretePulseGenerator  PulseType=Time based  Amplitude=-E_VEN * 0.99  Period=10000  PulseWidth=99  PhaseDelay=100
  Resistance3 : Subsystem
  V_VEN : Outport
  Q_VEN : Outport  Port=2
  tag scope: P_VEN=global
  wires:
  Add2/1 -> Resistance3/1(Pin), [P_VEN]  "P_VEN"
  Add/1 -> Add4/2, V_VEN/1
  Constant/1 -> Add/2
  Q_CSF/1 -> Add1/2
  Product/1 -> Add2/2
  Add1/1 -> Multiply/1
  Constant1/1 -> Add4/1
  Add4/1 -> Product/1
  Injection/1 -> Add1/1
  Integrator2/1 -> Add/1
  Constant5/1 -> Add3/1
  [P_ECS] -> Add2/1
  Multiply/1 -> Integrator2/1
  Add3/1 -> Product/2
  P_CMC/1 -> Resistance3/2(Pout)
  Resistance3/1(Q) -> Q_VEN/1, Add1/3
  Constant2/1 -> Resistance3/3(R)

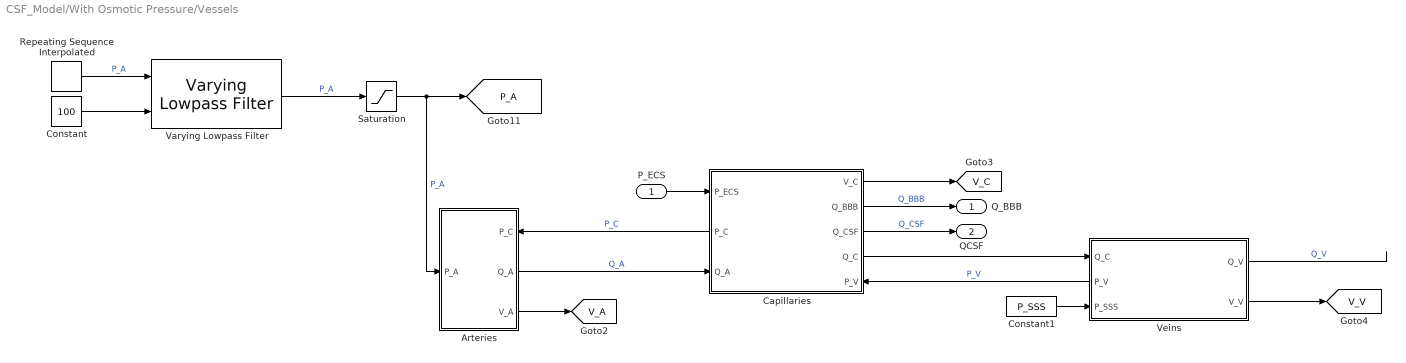
== system CSF_Model/With Osmotic Pressure/Vessels ==
  P_ECS : Inport
  Arteries : Subsystem
      settings: PortSchema="{\"entries\":[{\"content\":{\"sides\":[{\"content\":{\"connectorIds\":[\"In1\"]},\"type\":\"ConnectorPlacement.EquallySpacedRectSide\",\"uuid\":\"c8e2ba6b-712d-4498-a0c6-c2be4f5808b6\"},{\"content\":{\"connectorIds\":[\"In2\",\"Out1\",\"Out2\"],\"side\":\"RIGHT\"},\"type\":\"ConnectorPlacement.EquallySpacedRectSide\",\"uuid\":\"217d0c6f-0229-40b1-b57d-fa933108b642\"},{\"content\":{\"connectorIds\":[],\"side\":\"TOP\"},\"type\":\"ConnectorPlacement.EquallySpacedRectSide\",\"uuid\":\"a5a7b212-091d-4f85-aed6-99231843f7a9\"}]},\"type\":\"ConnectorPlacement.EquallySpacedConnector\",\"uuid\":\"228711f2-d096-4da2-871c-00d70df237bb\"}],\"packageUris\":[\"http://schema.mathworks.com/mf0/Connector/R2020b\"],\"version\":\"1.0\"}"
  Capillaries : Subsystem
      settings: PortSchema="{\"entries\":[{\"content\":{\"sides\":[{\"content\":{\"connectorIds\":[\"In1\",\"Out5\",\"In2\"]},\"type\":\"ConnectorPlacement.EquallySpacedRectSide\",\"uuid\":\"a84e4221-f33a-4452-85d5-f47e814dea9d\"},{\"content\":{\"connectorIds\":[\"Out1\",\"Out2\",\"Out3\",\"Out4\",\"In3\"],\"side\":\"RIGHT\"},\"type\":\"ConnectorPlacement.EquallySpacedRectSide\",\"uuid\":\"af720201-ea45-441f-b3d4-bc3a0b33f8d8\"},{\"content\":{\"connectorIds\":[],\"side\":\"TOP\"},\"type\":\"ConnectorPlacement.EquallySpacedRectSide\",\"uuid\":\"924ced81-9841-4533-ab32-ef11bc5e035f\"}]},\"type\":\"ConnectorPlacement.EquallySpacedConnector\",\"uuid\":\"f080819d-3a90-4942-8fa8-532e3452af47\"}],\"packageUris\":[\"http://schema.mathworks.com/mf0/Connector/R2020b\"],\"version\":\"1.0\"}"
  Constant : Constant  Value=100
  Constant1 : Constant  Value=P_SSS
  Repeating Sequence Interpolated : simulink/Sources/Repeating Sequence Interpolated  OutValues=central_cycle  TimeValues=t_fit  LookUpMeth=Use Input Nearest  tsamp=0.01  OutMin=[]  OutMax=[]  OutDataTypeStr=double  OutputDataTypeScalingMode=double  OutDataType=fixdt(0,8)  OutScaling=2^-10
  Saturation : Saturate  UpperLimit=200  LowerLimit=80
  Varying Lowpass Filter : cstblocks/Linear Parameter Varying/Varying Lowpass Filter  N=1
  Veins : Subsystem
      settings: PortSchema="{\"entries\":[{\"content\":{\"sides\":[{\"content\":{\"connectorIds\":[\"In1\",\"Out3\",\"In2\"]},\"type\":\"ConnectorPlacement.EquallySpacedRectSide\",\"uuid\":\"5b52797c-7783-4457-a0a9-3476d67ef718\"},{\"content\":{\"connectorIds\":[\"Out1\",\"Out2\"],\"side\":\"RIGHT\"},\"type\":\"ConnectorPlacement.EquallySpacedRectSide\",\"uuid\":\"96c05f31-9125-4d2f-8815-dd143ea35703\"},{\"content\":{\"connectorIds\":[],\"side\":\"TOP\"},\"type\":\"ConnectorPlacement.EquallySpacedRectSide\",\"uuid\":\"6951daa0-0f28-4dac-b2d6-1e8be48d433a\"}]},\"type\":\"ConnectorPlacement.EquallySpacedConnector\",\"uuid\":\"a58031d0-3fd5-4651-9fc5-fb87d5562115\"}],\"packageUris\":[\"http://schema.mathworks.com/mf0/Connector/R2020b\"],\"version\":\"1.0\"}"
  Q_BBB : Outport
  QCSF : Outport  Port=2
  tag scope: P_A=global, V_A=global, V_C=global, V_V=global
  wires:
  Arteries/2(V_A) -> [V_A]
  Constant1/1 -> Veins/2(P_SSS)
  Capillaries/5(P_C) -> Arteries/2(P_C)  "P_C"
  Arteries/1(Q_A) -> Capillaries/2(Q_A)  "Q_A"
  Veins/3(P_V) -> Capillaries/3(P_V)  "P_V"
  Veins/1(Q_V) -> ?  "Q_V"
  Capillaries/1(V_C) -> [V_C]
  Veins/2(V_V) -> [V_V]
  Capillaries/4(Q_C) -> Veins/1(Q_C)
  P_ECS/1 -> Capillaries/1(P_ECS)
  Capillaries/2(Q_BBB) -> Q_BBB/1  "Q_BBB"
  Capillaries/3(Q_CSF) -> QCSF/1  "Q_CSF"
  Repeating Sequence Interpolated/1 -> Varying Lowpass Filter/1  "P_A"
  Varying Lowpass Filter/1 -> Saturation/1  "P_A"
  Constant/1 -> Varying Lowpass Filter/2
  Saturation/1 -> Arteries/1(P_A), [P_A]  "P_A"

== system CSF_Model/With Osmotic Pressure/CMC (Cerebellomedullary Cistern)/Resistance1 ==
  Pin : Inport
  Pout : Inport  Port=2
  R : Inport  Port=3
  Divide : Product  Inputs=*/
  Subtract1 : Sum  Inputs=+-
  Q : Outport
  wires:
  Subtract1/1 -> Divide/1
  Pout/1 -> Subtract1/2
  Divide/1 -> Q/1
  Pin/1 -> Subtract1/1
  R/1 -> Divide/2

== system CSF_Model/With Osmotic Pressure/CMC (Cerebellomedullary Cistern)/Resistance2 ==
  Pin : Inport
  Pout : Inport  Port=2
  R : Inport  Port=3
  Divide : Product  Inputs=*/
  Subtract1 : Sum  Inputs=+-
  Q : Outport
  wires:
  R/1 -> Divide/2
  Pin/1 -> Subtract1/1
  Divide/1 -> Q/1
  Pout/1 -> Subtract1/2
  Subtract1/1 -> Divide/1

== system CSF_Model/With Osmotic Pressure/CMC (Cerebellomedullary Cistern)/Resistance3 ==
  Pin : Inport
  Pout : Inport  Port=2
  R : Inport  Port=3
  Divide : Product  Inputs=*/
  Subtract1 : Sum  Inputs=+-
  Q : Outport
  wires:
  R/1 -> Divide/2
  Pin/1 -> Subtract1/1
  Divide/1 -> Q/1
  Pout/1 -> Subtract1/2
  Subtract1/1 -> Divide/1

== system CSF_Model/With Osmotic Pressure/ECS/Resistance1 ==
  Pin : Inport
  Pout : Inport  Port=2
  R : Inport  Port=3
  Divide : Product  Inputs=*/
  Subtract1 : Sum  Inputs=+-
  Q : Outport
  wires:
  Subtract1/1 -> Divide/1
  Pout/1 -> Subtract1/2
  Divide/1 -> Q/1
  Pin/1 -> Subtract1/1
  R/1 -> Divide/2

== system CSF_Model/With Osmotic Pressure/ECS/Subsystem1 ==
  Signal Builder : Subsystem  Tag=STV Subsys  LoadFcn=sigbuilder_block('load');  StartFcn=sigbuilder_block('start');  StopFcn=sigbuilder_block('stop');  ClipboardFcn=sigbuilder_block('clipboard');  mask(Sigbuilder block){tuvar=[0:10]}
      mask help: Simulink:masks:SigbuilderBlock_MD
      mask init:
      | if ~strcmp(get_param(bdroot(gcbh),'SimulationStatus'),'stopped') tuvar = sigbuilder_block('maskInit'); end
      settings: CopyFcn=sigbuilder_block('copy');  DeleteFcn=sigbuilder_block('delete');  ModelCloseFcn=sigbuilder_block('modelClose');  PreSaveFcn=sigbuilder_block('preSave');  PauseFcn=sigbuilder_block('pause');  ContinueFcn=sigbuilder_block('continue');  NameChangeFcn=sigbuilder_block('namechange');  OpenFcn=sigbuilder_block('open',[324.75 228 550.5 399.75 ]);  CloseFcn=sigbuilder_block('close');
      mask Display: plot(0, 0, 100, 100,[2, 2, 32, 32, 2], [68, 8, 8, 68, 68],[32, 2], [38, 38], [32, 19, 2],[53, 60, 44], [32, 17, 17, 2],[16, 16, 31, 31]);txt = getActiveGroup(gcbh);text(2, 100, txt,'verticalAlignment', 'top');
  Out1 : Outport
  wires:
  Signal Builder/1(Signal 1) -> Out1/1

== system CSF_Model/With Osmotic Pressure/ICS/Resistance1 ==
  Pin : Inport
  Pout : Inport  Port=2
  R : Inport  Port=3
  Divide : Product  Inputs=*/
  Subtract1 : Sum  Inputs=+-
  Q : Outport
  wires:
  Subtract1/1 -> Divide/1
  Pout/1 -> Subtract1/2
  Divide/1 -> Q/1
  Pin/1 -> Subtract1/1
  R/1 -> Divide/2

== system CSF_Model/With Osmotic Pressure/PAS/Resistance2 ==
  Pin : Inport
  Pout : Inport  Port=2
  R : Inport  Port=3
  Divide : Product  Inputs=*/
  Subtract1 : Sum  Inputs=+-
  Q : Outport
  wires:
  Subtract1/1 -> Divide/1
  Pout/1 -> Subtract1/2
  Divide/1 -> Q/1
  Pin/1 -> Subtract1/1
  R/1 -> Divide/2

== system CSF_Model/With Osmotic Pressure/PAS/Resistance3 ==
  Pin : Inport
  Pout : Inport  Port=2
  R : Inport  Port=3
  Divide : Product  Inputs=*/
  Subtract1 : Sum  Inputs=+-
  Q : Outport
  wires:
  R/1 -> Divide/2
  Pin/1 -> Subtract1/1
  Divide/1 -> Q/1
  Pout/1 -> Subtract1/2
  Subtract1/1 -> Divide/1

== system CSF_Model/With Osmotic Pressure/SAS/Resistance1 ==
  Pin : Inport
  Pout : Inport  Port=2
  R : Inport  Port=3
  Divide : Product  Inputs=*/
  Subtract1 : Sum  Inputs=+-
  Q : Outport
  wires:
  Subtract1/1 -> Divide/1
  Pout/1 -> Subtract1/2
  Divide/1 -> Q/1
  Pin/1 -> Subtract1/1
  R/1 -> Divide/2

== system CSF_Model/With Osmotic Pressure/SAS/Resistance3 ==
  Pin : Inport
  Pout : Inport  Port=2
  R : Inport  Port=3
  Divide : Product  Inputs=*/
  Subtract1 : Sum  Inputs=+-
  Q : Outport
  wires:
  R/1 -> Divide/2
  Pin/1 -> Subtract1/1
  Divide/1 -> Q/1
  Pout/1 -> Subtract1/2
  Subtract1/1 -> Divide/1

== system CSF_Model/With Osmotic Pressure/SASE/Resistance1 ==
  Pin : Inport
  Pout : Inport  Port=2
  R : Inport  Port=3
  Divide : Product  Inputs=*/
  Subtract1 : Sum  Inputs=+-
  Q : Outport
  wires:
  Subtract1/1 -> Divide/1
  Pout/1 -> Subtract1/2
  Divide/1 -> Q/1
  Pin/1 -> Subtract1/1
  R/1 -> Divide/2

== system CSF_Model/With Osmotic Pressure/SASE/Resistance3 ==
  Pin : Inport
  Pout : Inport  Port=2
  R : Inport  Port=3
  Divide : Product  Inputs=*/
  Subtract1 : Sum  Inputs=+-
  Q : Outport
  wires:
  R/1 -> Divide/2
  Pin/1 -> Subtract1/1
  Divide/1 -> Q/1
  Pout/1 -> Subtract1/2
  Subtract1/1 -> Divide/1

== system CSF_Model/With Osmotic Pressure/Spinal SAS/Resistance1 ==
  Pin : Inport
  Pout : Inport  Port=2
  R : Inport  Port=3
  Divide : Product  Inputs=*/
  Subtract1 : Sum  Inputs=+-
  Q : Outport
  wires:
  Subtract1/1 -> Divide/1
  Pout/1 -> Subtract1/2
  Divide/1 -> Q/1
  Pin/1 -> Subtract1/1
  R/1 -> Divide/2

== system CSF_Model/With Osmotic Pressure/Subsystem1/Signal Builder ==
  Demux : Demux  Tag=STV Demux  Outputs=1
      settings: DisplayOption=none
  FromWs : FromWorkspace  Tag=STV FromWs  VariableName=tuvar
      SigBuilderData=|
      | common.afterFinalStr = 'Extrapolate'
      | common.sampleTime = 0
      | dataSet.timeRange = [0 100]
      | dataSet.name = 'Group 1'
      | sbobj.Groups.Name = 'Group 1'
      | sbobj.Groups.Signals.Name = 'Signal 1'
      | sbobj.Groups.Signals.XData = [0 35 35 40 40 100]
      | sbobj.Groups.Signals.YData = [0 0 300 300 0 0]
      | sbobj.Groups.TimeRange = [0 100]
  Signal 1 : Outport  Tag=STV Outport
  wires:
  Demux/1 -> Signal 1/1
  FromWs/1 -> Demux/1

== system CSF_Model/With Osmotic Pressure/Subsystem2/Signal Builder ==
  Demux : Demux  Tag=STV Demux  Outputs=1
      settings: DisplayOption=none
  FromWs : FromWorkspace  Tag=STV FromWs  VariableName=tuvar
      SigBuilderData=|
      | common.afterFinalStr = 'Extrapolate'
      | common.sampleTime = 0
      | dataSet.timeRange = [0 100]
      | dataSet.name = 'Group 1'
      | sbobj.Groups.Name = 'Group 1'
      | sbobj.Groups.Signals.Name = 'Signal 1'
      | sbobj.Groups.Signals.XData = [0 30.6 36.2 51.6 62.2 100]
      | sbobj.Groups.Signals.YData = [0 0 1.98 1.96 0.005 0]
      | sbobj.Groups.TimeRange = [0 100]
  Signal 1 : Outport  Tag=STV Outport
  wires:
  FromWs/1 -> Demux/1
  Demux/1 -> Signal 1/1

== system CSF_Model/With Osmotic Pressure/Subsystem3/Signal Builder ==
  Demux : Demux  Tag=STV Demux  Outputs=1
      settings: DisplayOption=none
  FromWs : FromWorkspace  Tag=STV FromWs  VariableName=tuvar
      SigBuilderData=|
      | common.afterFinalStr = 'Extrapolate'
      | common.sampleTime = 0
      | dataSet.timeRange = [0 10000]
      | dataSet.name = 'Group 1'
      | sbobj.Groups.Name = 'Group 1'
      | sbobj.Groups.Signals.Name = 'Signal 1'
      | sbobj.Groups.Signals.XData = [0 100 100 2100 2100 10000]
      | sbobj.Groups.Signals.YData = [0 0 1.5 1.5 0 0]
      | sbobj.Groups.TimeRange = [0 10000]
  Signal 1 : Outport  Tag=STV Outport
  wires:
  FromWs/1 -> Demux/1
  Demux/1 -> Signal 1/1

== system CSF_Model/With Osmotic Pressure/Subsystem4/Signal Builder ==
  Demux : Demux  Tag=STV Demux  Outputs=1
      settings: DisplayOption=none
  FromWs : FromWorkspace  Tag=STV FromWs  VariableName=tuvar
      SigBuilderData=|
      | common.afterFinalStr = 'Extrapolate'
      | common.sampleTime = 0
      | dataSet.timeRange = [0 100]
      | dataSet.name = 'Group 1'
      | sbobj.Groups.Name = 'Group 1'
      | sbobj.Groups.Signals.Name = 'Signal 1'
      | sbobj.Groups.Signals.XData = [0 35 35 40 40 100]
      | sbobj.Groups.Signals.YData = [0 0 300 300 0 0]
      | sbobj.Groups.TimeRange = [0 100]
  Signal 1 : Outport  Tag=STV Outport
  wires:
  Demux/1 -> Signal 1/1
  FromWs/1 -> Demux/1

== system CSF_Model/With Osmotic Pressure/Ventricles/Resistance3 ==
  Pin : Inport
  Pout : Inport  Port=2
  R : Inport  Port=3
  Divide : Product  Inputs=*/
  Subtract1 : Sum  Inputs=+-
  Q : Outport
  wires:
  R/1 -> Divide/2
  Pin/1 -> Subtract1/1
  Divide/1 -> Q/1
  Pout/1 -> Subtract1/2
  Subtract1/1 -> Divide/1

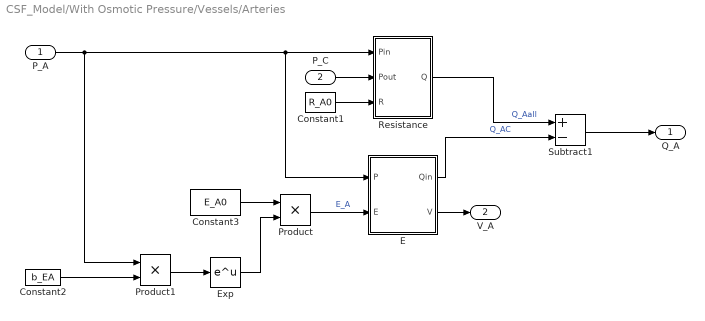
== system CSF_Model/With Osmotic Pressure/Vessels/Arteries ==
  P_A : Inport
  P_C : Inport  Port=2
  Constant1 : Constant  Value=R_A0
  Constant2 : Constant  Value=b_EA
  Constant3 : Constant  Value=E_A0
  E : Subsystem
  Exp : Math
  Product : Product
  Product1 : Product
  Resistance : Subsystem
  Subtract1 : Sum  Inputs=+-
  Q_A : Outport
  V_A : Outport  Port=2
  wires:
  Constant3/1 -> Product/1
  Constant1/1 -> Resistance/3(R)
  Resistance/1(Q) -> Subtract1/1  "Q_Aall"
  E/2(V) -> V_A/1
  E/1(Qin) -> Subtract1/2  "Q_AC"
  Subtract1/1 -> Q_A/1
  P_A/1 -> Product1/1, E/1(P), Resistance/1(Pin)
  P_C/1 -> Resistance/2(Pout)
  Exp/1 -> Product/2
  Constant2/1 -> Product1/2
  Product1/1 -> Exp/1
  Product/1 -> E/2(E)  "E_A"

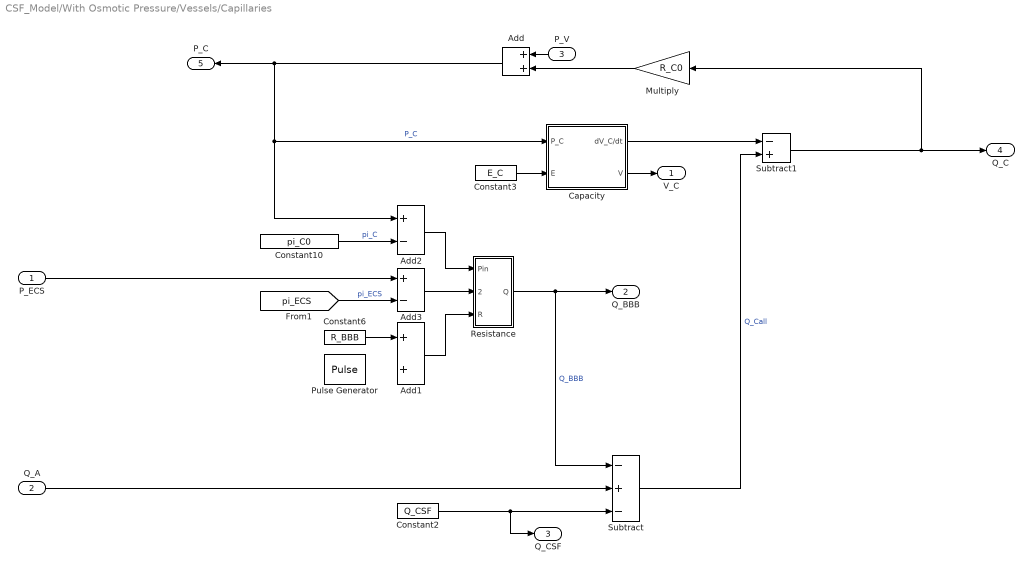
== system CSF_Model/With Osmotic Pressure/Vessels/Capillaries ==
  P_ECS : Inport
  Q_A : Inport  Port=2
  P_V : Inport  Port=3
  Add : Sum
  Add1 : Sum
  Add2 : Sum  Inputs=+-
  Add3 : Sum  Inputs=+-
  Capacity : Subsystem
  Constant10 : Constant  Value=pi_C0
  Constant2 : Constant  Value=Q_CSF
  Constant3 : Constant  Value=E_C
  Constant6 : Constant  Value=R_BBB
  Multiply : Gain  Gain=R_C0
  Pulse Generator : DiscretePulseGenerator  PulseType=Time based  Amplitude=-0.9*R_BBB  Period=1000  PulseWidth=10  PhaseDelay=50
  Resistance : Subsystem
  Subtract : Sum  Inputs=-+-
  Subtract1 : Sum  Inputs=-+
  V_C : Outport
  Q_BBB : Outport  Port=2
  Q_CSF : Outport  Port=3
  Q_C : Outport  Port=4
  P_C : Outport  Port=5
  wires:
  Constant3/1 -> Capacity/2(E)
  Add1/1 -> Resistance/3(R)
  Constant6/1 -> Add1/1
  Subtract/1 -> Subtract1/2  "Q_Call"
  Capacity/2(V) -> V_C/1
  Capacity/1(dV_C/dt) -> Subtract1/1
  Subtract1/1 -> Multiply/1, Q_C/1
  P_V/1 -> Add/1
  Add/1 -> Add2/1, Capacity/1(P_C), P_C/1  "P_C"
  Multiply/1 -> Add/2
  P_ECS/1 -> Add3/1
  Resistance/1(Q) -> Q_BBB/1, Subtract/1  "Q_BBB"
  Q_A/1 -> Subtract/2
  Add2/1 -> Resistance/1(Pin)
  Add3/1 -> Resistance/2(Pout)
  [pi_ECS] -> Add3/2  "pi_ECS"
  Constant10/1 -> Add2/2  "pi_C"
  Constant2/1 -> Q_CSF/1, Subtract/3

== system CSF_Model/With Osmotic Pressure/Vessels/Veins ==
  Q_C : Inport
  P_SSS : Inport  Port=2
  Add1 : Sum
  Constant3 : Constant  Value=E_V
  E : Subsystem
  Multiply2 : Gain  Gain=R_V0
  Subtract1 : Sum  Inputs=+-
  Q_V : Outport
  V_V : Outport  Port=2
  P_V : Outport  Port=3
  wires:
  E/2(V) -> V_V/1
  E/1(Qin) -> Subtract1/2
  Constant3/1 -> E/2(E)
  Add1/1 -> P_V/1, E/1(P)
  Multiply2/1 -> Add1/1
  Q_C/1 -> Subtract1/1
  P_SSS/1 -> Add1/2
  Subtract1/1 -> Q_V/1, Multiply2/1

== system CSF_Model/With Osmotic Pressure/ECS/Subsystem1/Signal Builder ==
  Demux : Demux  Tag=STV Demux  Outputs=1
      settings: DisplayOption=none
  FromWs : FromWorkspace  Tag=STV FromWs  VariableName=tuvar
      SigBuilderData=|
      | common.afterFinalStr = 'Extrapolate'
      | common.sampleTime = 0
      | dataSet.timeRange = [0 200]
      | dataSet.name = 'Group 1'
      | sbobj.Groups.Name = 'Group 1'
      | sbobj.Groups.Signals.Name = 'Signal 1'
      | sbobj.Groups.Signals.XData = [0 78.5 86 134 140 200]
      | sbobj.Groups.Signals.YData = [0 0 -0.294 -0.294 0 0]
      | sbobj.Groups.TimeRange = [0 200]
  Signal 1 : Outport  Tag=STV Outport
  wires:
  Demux/1 -> Signal 1/1
  FromWs/1 -> Demux/1

== system CSF_Model/With Osmotic Pressure/Vessels/Arteries/E ==
  P : Inport
  E : Inport  Port=2
  Add : Sum
  Constant2 : Constant  Value=V_Afree
  Derivative : Derivative
  Divide : Product  Inputs=*/
  Multiply : Gain  Gain=60
  Subtract2 : Sum  Inputs=+-
  Qin : Outport
  V : Outport  Port=2
  wires:
  Add/1 -> V/1  "V_A"
  Divide/1 -> Derivative/1, Add/1
  P/1 -> Subtract2/1
  Derivative/1 -> Multiply/1  "Q_AC"
  Subtract2/1 -> Divide/1
  E/1 -> Divide/2
  Constant2/1 -> Add/2
  [P_ECS] -> Subtract2/2
  Multiply/1 -> Qin/1

== system CSF_Model/With Osmotic Pressure/Vessels/Arteries/Resistance ==
  Pin : Inport
  Pout : Inport  Port=2
  R : Inport  Port=3
  Divide : Product  Inputs=*/
  Subtract1 : Sum  Inputs=+-
  Q : Outport
  wires:
  R/1 -> Divide/2
  Pin/1 -> Subtract1/1
  Divide/1 -> Q/1
  Pout/1 -> Subtract1/2
  Subtract1/1 -> Divide/1

== system CSF_Model/With Osmotic Pressure/Vessels/Capillaries/Capacity ==
  P_C : Inport
  E : Inport  Port=2
  Add : Sum
  Constant2 : Constant  Value=V_Cfree
  Derivative : Derivative
  Divide : Product  Inputs=*/
  Multiply : Gain  Gain=60
  Subtract2 : Sum  Inputs=+-
  dV_C/dt : Outport
  V : Outport  Port=2
  wires:
  Add/1 -> V/1
  Divide/1 -> Derivative/1, Add/1
  P_C/1 -> Subtract2/1
  Derivative/1 -> Multiply/1
  Subtract2/1 -> Divide/1
  [P_ECS] -> Subtract2/2
  E/1 -> Divide/2
  Constant2/1 -> Add/2
  Multiply/1 -> dV_C/dt/1

== system CSF_Model/With Osmotic Pressure/Vessels/Capillaries/Resistance ==
  Pin : Inport
  Pout : Inport  Port=2
  R : Inport  Port=3
  Divide : Product  Inputs=*/
  Subtract1 : Sum  Inputs=+-
  Q : Outport
  wires:
  R/1 -> Divide/2
  Pin/1 -> Subtract1/1
  Divide/1 -> Q/1
  Pout/1 -> Subtract1/2
  Subtract1/1 -> Divide/1

== system CSF_Model/With Osmotic Pressure/Vessels/Veins/E ==
  P : Inport
  E : Inport  Port=2
  Add : Sum
  Constant2 : Constant  Value=V_Vfree
  Derivative : Derivative
  Divide : Product  Inputs=*/
  Multiply : Gain  Gain=60
  Subtract : Sum  Inputs=+-
  Qin : Outport
  V : Outport  Port=2
  wires:
  E/1 -> Divide/2
  Add/1 -> V/1
  Divide/1 -> Multiply/1, Add/1
  Derivative/1 -> Qin/1  "Q_C"
  Subtract/1 -> Divide/1
  P/1 -> Subtract/1
  [P_PNS] -> Subtract/2
  Constant2/1 -> Add/2
  Multiply/1 -> Derivative/1
